simulink model "Computed_Torque_FwdControl"  (Simulink 7.9)
settings: Solver=ode45  StartTime=0.0  StopTime=10.0  RelTol=1e-3
undefined symbols (not defined in the file): AccLimit, AccSourceSelect, DiscIntNeverNeededParam, KA, km, KP, kt, kTA, kTP, kTV, KV, LinePTs2Rpm, PosSourceSelect, Ra, TA, TauLimit, Ts, VelLimit, VelSourceSelect
libraries: powerlib_extras x6
settings Model: Creator=Administrator  LastModifiedBy=Administrator

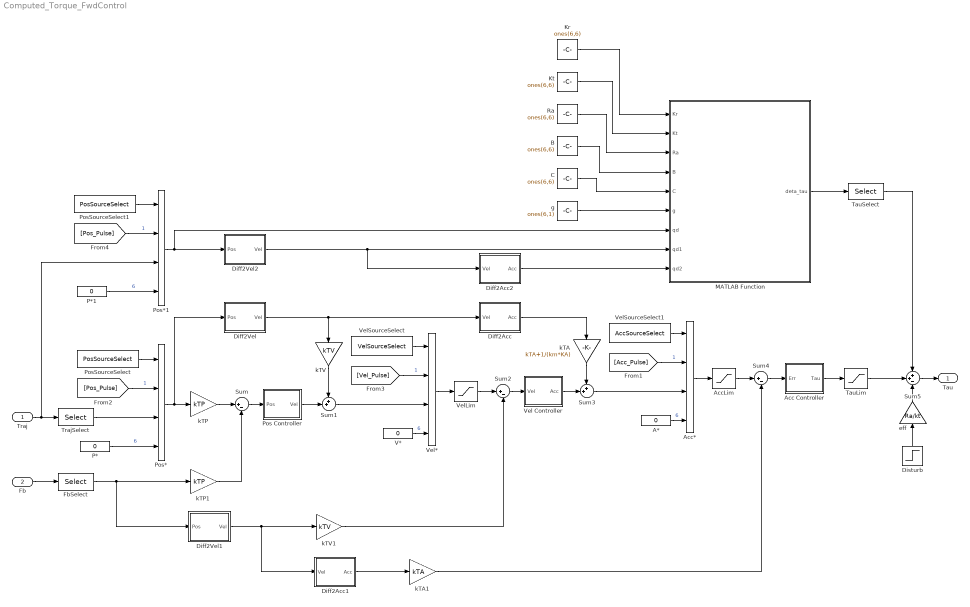
== system Computed_Torque_FwdControl ==
  Traj : Inport
  Fb : Inport  Port=2
  A* : Constant  Value=0  SampleTime=Ts
  Acc Controller : Subsystem
  Acc* : MultiPortSwitch  zeroidx=off
  AccLim : Saturate  UpperLimit=AccLimit  LowerLimit=-AccLimit  SampleTime=Ts
  B : Constant  Value=ones(6,6)
  C : Constant  Value=ones(6,6)
  Diff2Acc : Subsystem
  Diff2Acc1 : Subsystem
  Diff2Acc2 : Subsystem
  Diff2Vel : Subsystem
  Diff2Vel1 : Subsystem
  Diff2Vel2 : Subsystem
  Disturb : Step  SampleTime=0
  FbSelect : Selector  InputPortWidth=6  IndexOptions=Index vector (dialog)  Indices=AxisNO  OutputSizes=1
  Kr : Constant  Value=ones(6,6)
  Kt : Constant  Value=ones(6,6)
  MATLAB Function : MATLAB Function  TreatAsAtomicUnit=on
  P* : Constant  Value=0  SampleTime=Ts
  P*1 : Constant  Value=0  SampleTime=Ts
  Pos Controller : Subsystem
  Pos* : MultiPortSwitch  zeroidx=off  SampleTime=Ts
  Pos*1 : MultiPortSwitch  zeroidx=off  SampleTime=Ts
  PosSourceSelect : Constant  Value=PosSourceSelect  SampleTime=Ts
  PosSourceSelect1 : Constant  Value=PosSourceSelect  SampleTime=Ts
  Ra : Constant  Value=ones(6,6)
  Sum : Sum  Inputs=|+-  SampleTime=Ts
  Sum1 : Sum  Inputs=++|  SampleTime=Ts
  Sum2 : Sum  Inputs=|+-  SampleTime=Ts
  Sum3 : Sum  Inputs=++|  SampleTime=Ts
  Sum4 : Sum  Inputs=|+-  SampleTime=Ts
  Sum5 : Sum  Inputs=++-  SampleTime=Ts
  TauLim : Saturate  UpperLimit=TauLimit  LowerLimit=-TauLimit  SampleTime=Ts
  TauSelect : Selector  InputPortWidth=6  IndexOptions=Index vector (dialog)  Indices=AxisNO  OutputSizes=1
  TrajSelect : Selector  InputPortWidth=6  IndexOptions=Index vector (dialog)  Indices=AxisNO  OutputSizes=1
  V* : Constant  Value=0  SampleTime=Ts
  Vel Controller : Subsystem
  Vel* : MultiPortSwitch  zeroidx=off
  VelLim : Saturate  UpperLimit=VelLimit  LowerLimit=-VelLimit  SampleTime=Ts
  VelSourceSelect : Constant  Value=VelSourceSelect  SampleTime=Ts
  VelSourceSelect1 : Constant  Value=AccSourceSelect  SampleTime=Ts
  eff : Gain  Gain=Ra/kt  SampleTime=Ts
  g : Constant  Value=ones(6,1)
  kTA : Gain  Gain=kTA+1/(km*KA)  SampleTime=Ts
  kTA1 : Gain  Gain=kTA  SampleTime=Ts
  kTP : Gain  Gain=kTP  SampleTime=Ts
  kTP1 : Gain  Gain=kTP  SampleTime=Ts
  kTV : Gain  Gain=kTV  SampleTime=Ts
  kTV1 : Gain  Gain=kTV  SampleTime=Ts
  Tau : Outport
  wires:
  [Pos_Pulse] -> Pos*/2  "1"
  TrajSelect/1 -> Pos*/3
  P*/1 -> Pos*/4  "6"
  PosSourceSelect/1 -> Pos*/1
  Traj/1 -> TrajSelect/1, Pos*1/3
  Pos*/1 -> kTP/1, Diff2Vel/1(Pos)
  kTP/1 -> Sum/1
  Sum/1 -> Pos Controller/1(Pos)
  Pos Controller/1(Vel) -> Sum1/2
  kTV/1 -> Sum1/1
  Diff2Vel/1(Vel) -> kTV/1, Diff2Acc/1(Vel)
  VelLim/1 -> Sum2/1
  Vel Controller/1(Acc) -> Sum3/2
  Diff2Acc/1(Acc) -> kTA/1
  kTA/1 -> Sum3/1
  V*/1 -> Vel*/4  "6"
  [Vel_Pulse] -> Vel*/2  "1"
  Vel*/1 -> VelLim/1
  VelSourceSelect/1 -> Vel*/1
  Sum1/1 -> Vel*/3
  AccLim/1 -> Sum4/1
  Sum4/1 -> Acc Controller/1(Err)
  Sum2/1 -> Vel Controller/1(Vel)
  Acc Controller/1(Tau) -> TauLim/1
  Sum5/1 -> Tau/1
  Fb/1 -> FbSelect/1
  FbSelect/1 -> kTP1/1, Diff2Vel1/1(Pos)
  kTP1/1 -> Sum/2
  Diff2Vel1/1(Vel) -> kTV1/1, Diff2Acc1/1(Vel)
  kTV1/1 -> Sum2/2
  Diff2Acc1/1(Acc) -> kTA1/1
  kTA1/1 -> Sum4/2
  A*/1 -> Acc*/4  "6"
  [Acc_Pulse] -> Acc*/2  "1"
  VelSourceSelect1/1 -> Acc*/1
  Sum3/1 -> Acc*/3
  Acc*/1 -> AccLim/1
  TauLim/1 -> Sum5/2
  eff/1 -> Sum5/3
  Disturb/1 -> eff/1
  Diff2Vel2/1(Vel) -> MATLAB Function/8(qd1), Diff2Acc2/1(Vel)
  Diff2Acc2/1(Acc) -> MATLAB Function/9(qd2)
  [Pos_Pulse] -> Pos*1/2  "1"
  P*1/1 -> Pos*1/4  "6"
  PosSourceSelect1/1 -> Pos*1/1
  Pos*1/1 -> Diff2Vel2/1(Pos), MATLAB Function/7(qd)
  Kr/1 -> MATLAB Function/1(Kr)
  Kt/1 -> MATLAB Function/2(Kt)
  g/1 -> MATLAB Function/6(g)
  C/1 -> MATLAB Function/5(C)
  B/1 -> MATLAB Function/4(B)
  Ra/1 -> MATLAB Function/3(Ra)
  MATLAB Function/1(deta_tau) -> TauSelect/1
  TauSelect/1 -> Sum5/1

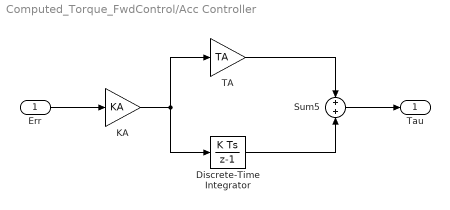
== system Computed_Torque_FwdControl/Acc Controller ==
  Err : Inport
  Discrete-Time Integrator : DiscreteIntegrator  SampleTime=Ts  ICPrevOutput=DiscIntNeverNeededParam  ICPrevScaledInput=DiscIntNeverNeededParam
  KA : Gain  Gain=KA  SampleTime=Ts
  Sum5 : Sum  Inputs=+|+
  TA : Gain  Gain=TA  SampleTime=Ts
  Tau : Outport
  wires:
  TA/1 -> Sum5/1
  Discrete-Time Integrator/1 -> Sum5/2
  KA/1 -> TA/1, Discrete-Time Integrator/1
  Err/1 -> KA/1
  Sum5/1 -> Tau/1

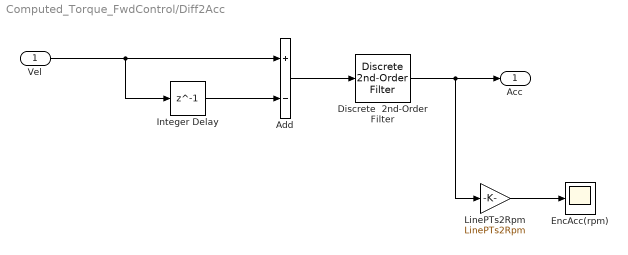
== system Computed_Torque_FwdControl/Diff2Acc ==
  Vel : Inport
  Add : Sum  Inputs=+-
  Discrete  2nd-Order Filter : powerlib_extras/Discrete  Control Blocks/Discrete  2nd-Order Filter  FilterType=Lowpass  Fo=200  Zeta=0.707  Ts=Ts  Initialize=off  Vac_Init=[0.8 -25 60]  Vdc_Init=-0.4  PlotResponse=off  param1=[1 5000 10]
  EncAcc(rpm) : Scope
      settings: SaveName=ScopeData33
  Integer Delay : Delay  DelayLength=1  InputProcessing=Inherited
  LinePTs2Rpm : Gain  Gain=LinePTs2Rpm
  Acc : Outport
  wires:
  Add/1 -> Discrete  2nd-Order Filter/1
  Discrete  2nd-Order Filter/1 -> Acc/1, LinePTs2Rpm/1
  Vel/1 -> Integer Delay/1, Add/1
  Integer Delay/1 -> Add/2
  LinePTs2Rpm/1 -> EncAcc(rpm)/1

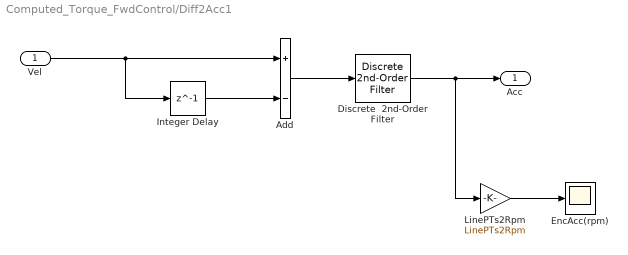
== system Computed_Torque_FwdControl/Diff2Acc1 ==
  Vel : Inport
  Add : Sum  Inputs=+-
  Discrete  2nd-Order Filter : powerlib_extras/Discrete  Control Blocks/Discrete  2nd-Order Filter  FilterType=Lowpass  Fo=200  Zeta=0.707  Ts=Ts  Initialize=off  Vac_Init=[0.8 -25 60]  Vdc_Init=-0.4  PlotResponse=off  param1=[1 5000 10]
  EncAcc(rpm) : Scope
      settings: SaveName=ScopeData33
  Integer Delay : Delay  DelayLength=1  InputProcessing=Inherited
  LinePTs2Rpm : Gain  Gain=LinePTs2Rpm
  Acc : Outport
  wires:
  Add/1 -> Discrete  2nd-Order Filter/1
  Discrete  2nd-Order Filter/1 -> Acc/1, LinePTs2Rpm/1
  Vel/1 -> Integer Delay/1, Add/1
  Integer Delay/1 -> Add/2
  LinePTs2Rpm/1 -> EncAcc(rpm)/1

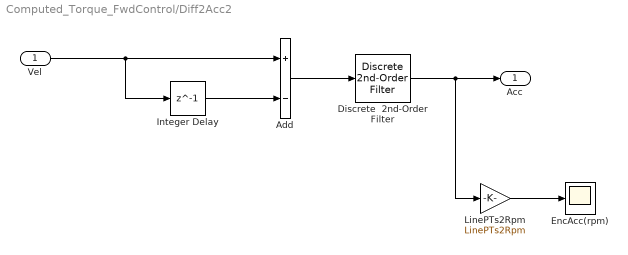
== system Computed_Torque_FwdControl/Diff2Acc2 ==
  Vel : Inport
  Add : Sum  Inputs=+-
  Discrete  2nd-Order Filter : powerlib_extras/Discrete  Control Blocks/Discrete  2nd-Order Filter  FilterType=Lowpass  Fo=200  Zeta=0.707  Ts=Ts  Initialize=off  Vac_Init=[0.8 -25 60]  Vdc_Init=-0.4  PlotResponse=off  param1=[1 5000 10]
  EncAcc(rpm) : Scope
      settings: SaveName=ScopeData33
  Integer Delay : Delay  DelayLength=1  InputProcessing=Inherited
  LinePTs2Rpm : Gain  Gain=LinePTs2Rpm
  Acc : Outport
  wires:
  Add/1 -> Discrete  2nd-Order Filter/1
  Discrete  2nd-Order Filter/1 -> Acc/1, LinePTs2Rpm/1
  Vel/1 -> Integer Delay/1, Add/1
  Integer Delay/1 -> Add/2
  LinePTs2Rpm/1 -> EncAcc(rpm)/1

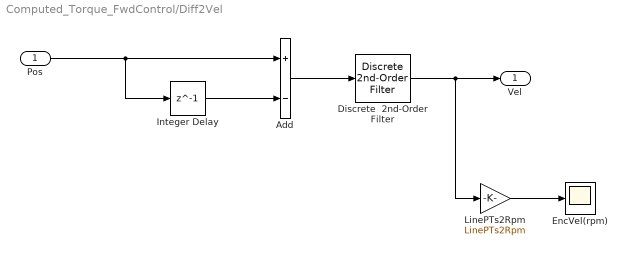
== system Computed_Torque_FwdControl/Diff2Vel ==
  Pos : Inport
  Add : Sum  Inputs=+-
  Discrete  2nd-Order Filter : powerlib_extras/Discrete  Control Blocks/Discrete  2nd-Order Filter  FilterType=Lowpass  Fo=200  Zeta=0.707  Ts=Ts  Initialize=off  Vac_Init=[0.8 -25 60]  Vdc_Init=-0.4  PlotResponse=off  param1=[1 5000 10]
  EncVel(rpm) : Scope
      settings: SaveName=ScopeData33
  Integer Delay : Delay  DelayLength=1  InputProcessing=Inherited
  LinePTs2Rpm : Gain  Gain=LinePTs2Rpm
  Vel : Outport
  wires:
  Add/1 -> Discrete  2nd-Order Filter/1
  Discrete  2nd-Order Filter/1 -> Vel/1, LinePTs2Rpm/1
  Pos/1 -> Integer Delay/1, Add/1
  Integer Delay/1 -> Add/2
  LinePTs2Rpm/1 -> EncVel(rpm)/1

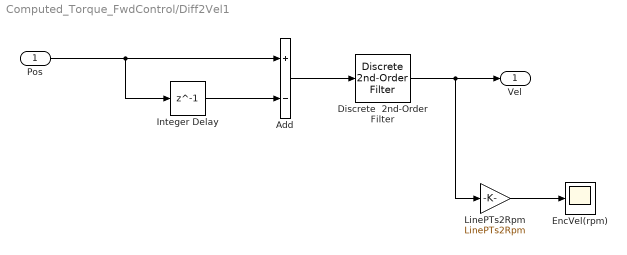
== system Computed_Torque_FwdControl/Diff2Vel1 ==
  Pos : Inport
  Add : Sum  Inputs=+-
  Discrete  2nd-Order Filter : powerlib_extras/Discrete  Control Blocks/Discrete  2nd-Order Filter  FilterType=Lowpass  Fo=200  Zeta=0.707  Ts=Ts  Initialize=off  Vac_Init=[0.8 -25 60]  Vdc_Init=-0.4  PlotResponse=off  param1=[1 5000 10]
  EncVel(rpm) : Scope
      settings: SaveName=ScopeData33
  Integer Delay : Delay  DelayLength=1  InputProcessing=Inherited
  LinePTs2Rpm : Gain  Gain=LinePTs2Rpm
  Vel : Outport
  wires:
  Add/1 -> Discrete  2nd-Order Filter/1
  Discrete  2nd-Order Filter/1 -> Vel/1, LinePTs2Rpm/1
  Pos/1 -> Integer Delay/1, Add/1
  Integer Delay/1 -> Add/2
  LinePTs2Rpm/1 -> EncVel(rpm)/1

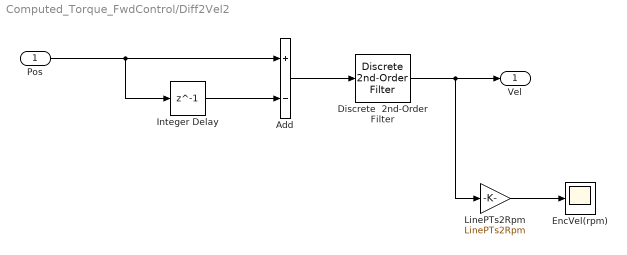
== system Computed_Torque_FwdControl/Diff2Vel2 ==
  Pos : Inport
  Add : Sum  Inputs=+-
  Discrete  2nd-Order Filter : powerlib_extras/Discrete  Control Blocks/Discrete  2nd-Order Filter  FilterType=Lowpass  Fo=200  Zeta=0.707  Ts=Ts  Initialize=off  Vac_Init=[0.8 -25 60]  Vdc_Init=-0.4  PlotResponse=off  param1=[1 5000 10]
  EncVel(rpm) : Scope
      settings: SaveName=ScopeData33
  Integer Delay : Delay  DelayLength=1  InputProcessing=Inherited
  LinePTs2Rpm : Gain  Gain=LinePTs2Rpm
  Vel : Outport
  wires:
  Add/1 -> Discrete  2nd-Order Filter/1
  Discrete  2nd-Order Filter/1 -> Vel/1, LinePTs2Rpm/1
  Pos/1 -> Integer Delay/1, Add/1
  Integer Delay/1 -> Add/2
  LinePTs2Rpm/1 -> EncVel(rpm)/1

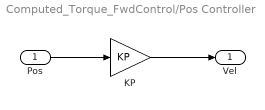
== system Computed_Torque_FwdControl/Pos Controller ==
  Pos : Inport
  KP : Gain  Gain=KP  SampleTime=Ts
  Vel : Outport
  wires:
  Pos/1 -> KP/1
  KP/1 -> Vel/1

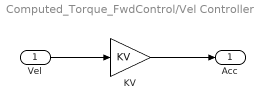
== system Computed_Torque_FwdControl/Vel Controller ==
  Vel : Inport
  KV : Gain  Gain=KV  SampleTime=Ts
  Acc : Outport
  wires:
  Vel/1 -> KV/1
  KV/1 -> Acc/1

== matlab function MATLAB Function ==
  data: Kr input double; Kt input double; Ra input double; B input double; C input double; g input double; qd input double; deta_tau output double; qd1 input double; qd2 input double
function deta_tau = ComputedTorque_Fwd(Kr,Kt,Ra,B,C,g,qd,qd1,qd2)
%#codegen
%qmd-pos qmd1-vel qmd2-acc
qmd=Kr*qd;
qmd1=Kr*qd1;
qmd2=Kr*qd2;
v=diag(B);
Bbar=diag(v,0);
detaB=B-Bbar;
dd=inv(Kr)*detaB*inv(Kr)*qmd2+inv(Kr)*C*inv(Kr)*qmd1+inv(Kr)*g;
deta_tau=Ra*inv(Kt)*dd;
end
